simulink model "callGAMS"  (R2021b)
settings: Solver=ode1  StartTime=0.0  StopTime=20  FixedStep=1e-4  RelTol=1e-3
model workspace (MAT data in the model file):
  firstOrder = 60
  g2Max = 0
  runTime = 4
undefined symbols (not defined in the file or in its folder): c0, c1, D11, Delta, fg, G2gen, G3gen, G5gen, G6gen, G7gen, Iovc, l0, l1, Newton, r0, r1, Raphson, Rtpu, S1non, S2non, S3non, S5non, S6non, S7non, sigbuilder_block, tonvsc, Ts, Vhv, Vmv, w_pll, wc1, wdc1, wpq1, wsw1, Xtpu
libraries: simulink_extras x122, simulink x73, spsFirstOrderFilterLib x72, spsGroundLib x61, spsCurrentMeasurementLib x33, spsVoltageMeasurementLib x33, eeTransforms x24, spsabctoAlphaBetaZeroLib x12, spsControlledVoltageSourceLib x12, spsControlledCurrentSourceLib x12, spsPower3phPhasorLib x11, spsLoadFlowBusLib x9
(part 4 of 16)

== system callGAMS/sm_computation/G1/Speed Governor ==
  note: mechanical power
  RefL : Inport
  dw : Inport  Port=2
  Gain1 : Gain  Gain=Dt
  Gain2 : Gain  Gain=1/R
  Saturation : Saturate  UpperLimit=Vmax  LowerLimit=Vmin
  Saturation1 : Saturate  UpperLimit=1
  Sum : Sum  Inputs=|+-
  Sum1 : Sum  Inputs=|+-
  Transfer Fcn (with initial outputs)1 : simulink_extras/Additional Linear/Transfer Fcn (with initial outputs)  N=[T2 1]  D=[T3 1]  Y0=P0  U0=P0
  Transfer Fcn (with initial outputs)2 : simulink_extras/Additional Linear/Transfer Fcn (with initial outputs)  N=[1]  D=[T1 1]  Y0=P0  U0=P0
  Pm : Outport
  wires:
  Saturation1/1 -> Pm/1
  RefL/1 -> Sum/1
  Sum/1 -> Transfer Fcn (with initial outputs)2/1
  Transfer Fcn (with initial outputs)2/1 -> Saturation/1
  Saturation/1 -> Transfer Fcn (with initial outputs)1/1
  Sum1/1 -> Saturation1/1
  Transfer Fcn (with initial outputs)1/1 -> Sum1/1
  Gain1/1 -> Sum1/2
  dw/1 -> Gain1/1, Gain2/1
  Gain2/1 -> Sum/2

== system callGAMS/sm_computation/G2/G2 setpoint ==
  Clock : Clock
      settings: Decimation=runTime
  Clock1 : Clock
  Clock2 : Clock
      settings: Decimation=runTime
  Constant1 : Constant  Value=S2non*G2gen
  Constant2 : Constant  Value=S2non*G2gen
  Gain : Gain  Gain=1e6/1.2
  Gain1 : Gain  Gain=1/120
  Integrator : Integrator  InitialCondition=S2non*G2gen
  Memory : Memory
  Min : MinMax  Inputs=2
  Min1 : MinMax  Function=max  Inputs=2
  Sum : Sum  Inputs=|+-
  Sum1 : Sum
  Sum2 : Sum
  Sum3 : Sum
  Switch : Switch  Criteria=u2 > Threshold  Threshold=1  InputSameDT=on
  Switch1 : Switch  Criteria=u2 > Threshold  Threshold=runTime+1
  Switch2 : Switch  Criteria=u2 > Threshold  Threshold=runTime
  Switch3 : Switch  InputSameDT=on
  Switch4 : Switch  Criteria=u2 > Threshold  Threshold=runTime
  Out1 : Outport
  tag scope: g2Actual=global, g2Expected=global
  wires:
  [g2] -> Switch2/1
  Clock1/1 -> Switch1/2
  Sum1/1 -> Switch1/1
  Memory/1 -> Sum1/1
  Clock/1 -> Switch2/2
  Constant2/1 -> Switch2/3
  Switch/1 -> ?
  Gain/1 -> Sum2/2
  Switch2/1 -> Sum2/1, [g2Actual], Switch1/3
  [g2Reg] -> Sum1/2
  [g2Reg] -> Gain/1
  Sum2/1 -> Min1/2, Min/2
  Switch1/1 -> Switch/2, Switch/3, [A], Memory/1
  [A] -> Min1/1, Min/1
  [gSet] -> Switch/1
  [g2Reg] -> Switch3/2
  Min/1 -> Switch3/1
  Min1/1 -> Switch3/3
  Switch3/1 -> [gSet]
  [g2] -> Sum3/1
  Constant1/1 -> Switch4/3
  Clock2/1 -> Switch4/2
  Sum3/1 -> Switch4/1
  [g2Reg] -> Sum3/2
  Switch4/1 -> [g2Expected], Sum/1
  Integrator/1 -> Out1/1, Sum/2
  Sum/1 -> Gain1/1
  Gain1/1 -> Integrator/1

== system callGAMS/sm_computation/G2/VSC v2 ==
  note: If using different transformer connection,
      | compensate the delay in the modulation
  Pset : Inport
  Qset : Inport  Port=2
  Block : Step  Time=tonvsc  Before=1  After=0  SampleTime=0
  NOT : Logic  Operator=NOT  IconShape=distinctive  AllPortsSameDT=off  OutDataTypeStr=boolean
  Three-Phase Transformer (Two Windings)1 : spsThreePhaseTransformerTwoWindingsLib/Three-Phase Transformer (Two Windings)  Winding1Connection=Yg  Winding2Connection=Delta (D11)  CoreType=Three single-phase transformers  SetSaturation=off  Hysteresis=off  DataFile='hysteresis'  SetInitialFlux=off  Measurements=None  UNITS=pu  NominalPower=[Pconv , fg]  Winding1=[Vhv, Rtpu/2, Xtpu/2]  Winding2=[Vmv, Rtpu/2, Xtpu/2]  Rm=5000  Lm=5000  L0=0.5  Saturation=[ 0,0 ; 0.0024,1.2 ; 1.0,1.52 ]  InitialFluxes=[ 0.8 , -0.8 , 0.7 ]  BreakLoop=off  DiscreteSolver=Trapezoidal iterative  DataType=off  TransfoNumber=1
  VI measurement : Subsystem
  VSC Control : Subsystem
  VSC Model : Subsystem  Variant=on  VariantControlMode=label  LabelModeActiveChoice=Phasor
  output signals : Subsystem
  A : PMIOPort  Side=Left
  B : PMIOPort  Port=2  Side=Left
  C : PMIOPort  Port=3  Side=Left
  m : Outport
  tag scope: I2=global, V2=global
  wires:
  NOT/1 -> ?
  VSC Control/1(Ref) -> VSC Model/1(Ref)
  [Is] -> VSC Control/3(Iabc)
  Block/1 -> NOT/1, VSC Control/1(Block)
  [Vs] -> output signals/1(Vs)
  [Is] -> output signals/2(Is)
  VSC Control/2(m) -> output signals/3(control)
  output signals/1(m) -> m/1
  VI measurement/1(Vs) -> [V2], [Vs]
  VI measurement/2(Is) -> [I2], [Is]
  Qset/1 -> VSC Control/5(Qset)
  [Vs] -> VSC Control/2(Vabc)
  Pset/1 -> VSC Control/4(Pset)
  ? -> VSC Control/6(Edc)
  connections:
  Three-Phase Transformer (Two Windings)1/LConn3 -- VI measurement/LConn3
  Three-Phase Transformer (Two Windings)1/LConn2 -- VI measurement/LConn2
  Three-Phase Transformer (Two Windings)1/LConn1 -- VI measurement/LConn1
  Three-Phase Transformer (Two Windings)1/RConn3 -- VSC Model/LConn3
  Three-Phase Transformer (Two Windings)1/RConn2 -- VSC Model/LConn2
  Three-Phase Transformer (Two Windings)1/RConn1 -- VSC Model/LConn1
  VI measurement/RConn1 -- A/RConn1
  VI measurement/RConn2 -- B/RConn1
  VI measurement/RConn3 -- C/RConn1

== system callGAMS/sm_computation/G3/G3 setpoint ==
  Clock : Clock
      settings: Decimation=runTime
  Clock1 : Clock
  Clock2 : Clock
      settings: Decimation=runTime
  Constant1 : Constant  Value=S3non*G3gen
  Constant2 : Constant  Value=S3non*G3gen
  Gain : Gain  Gain=1e6/1.2
  Gain1 : Gain  Gain=1/120
  Integrator : Integrator  InitialCondition=S2non*G2gen
  Memory : Memory
  Min : MinMax  Inputs=2
  Min1 : MinMax  Function=max  Inputs=2
  Sum : Sum  Inputs=|+-
  Sum1 : Sum
  Sum2 : Sum
  Sum3 : Sum
  Switch : Switch  Criteria=u2 > Threshold  Threshold=1  InputSameDT=on
  Switch1 : Switch  Criteria=u2 > Threshold  Threshold=runTime+1
  Switch2 : Switch  Criteria=u2 > Threshold  Threshold=runTime
  Switch3 : Switch  InputSameDT=on
  Switch4 : Switch  Criteria=u2 > Threshold  Threshold=runTime
  Out1 : Outport
  tag scope: g3Expected=global, g3toOpt=global
  wires:
  [g3] -> Switch2/1
  Clock1/1 -> Switch1/2
  Sum1/1 -> Switch1/1
  Memory/1 -> Sum1/1
  Clock/1 -> Switch2/2
  Constant2/1 -> Switch2/3
  Switch/1 -> Out1/1
  Gain/1 -> Sum2/2
  Switch2/1 -> Switch1/3, [g3toOpt], Sum2/1
  [g3Reg] -> Sum1/2
  [g3Reg] -> Gain/1
  Sum2/1 -> Min1/2, Min/2
  Switch1/1 -> Memory/1, [A], Switch/3, Switch/2
  [A] -> Min1/1, Min/1
  [gSet] -> Switch/1
  [g3Reg] -> Switch3/2
  Min/1 -> Switch3/1
  Min1/1 -> Switch3/3
  Switch3/1 -> [gSet]
  Gain1/1 -> Integrator/1
  Sum/1 -> Gain1/1
  Integrator/1 -> Sum/2
  Sum3/1 -> Switch4/1
  Constant1/1 -> Switch4/3
  Clock2/1 -> Switch4/2
  [g3] -> Sum3/1
  [g3Reg] -> Sum3/2
  Switch4/1 -> [g3Expected], Sum/1

== system callGAMS/sm_computation/G3/VSC v2 ==
  note: If using different transformer connection,
      | compensate the delay in the modulation
  Pset : Inport
  Qset : Inport  Port=2
  Block : Step  Time=tonvsc  Before=1  After=0  SampleTime=0
  NOT : Logic  Operator=NOT  IconShape=distinctive  AllPortsSameDT=off  OutDataTypeStr=boolean
  Three-Phase Transformer (Two Windings) : spsThreePhaseTransformerTwoWindingsLib/Three-Phase Transformer (Two Windings)  Winding1Connection=Yg  Winding2Connection=Delta (D11)  CoreType=Three single-phase transformers  SetSaturation=off  Hysteresis=off  DataFile='hysteresis'  SetInitialFlux=off  Measurements=None  UNITS=pu  NominalPower=[Pconv , fg ]  Winding1=[Vhv, Rtpu/2, Xtpu/2]  Winding2=[Vmv, Rtpu/2, Xtpu/2]  Rm=5000  Lm=5000  L0=0.5  Saturation=[ 0,0 ; 0.0024,1.2 ; 1.0,1.52 ]  InitialFluxes=[ 0.8 , -0.8 , 0.7 ]  BreakLoop=off  DiscreteSolver=Trapezoidal iterative  DataType=off  TransfoNumber=1
  VI measurement1 : Subsystem
  VSC Control : Subsystem
  VSC Model : Subsystem  Variant=on  VariantControlMode=label  LabelModeActiveChoice=Phasor
  output signals : Subsystem
  A : PMIOPort  Side=Left
  B : PMIOPort  Port=2  Side=Left
  C : PMIOPort  Port=3  Side=Left
  m : Outport
  tag scope: I3=global, V3=global
  wires:
  NOT/1 -> ?
  VSC Control/1(Ref) -> VSC Model/1(Ref)
  [Is] -> VSC Control/3(Iabc)
  Block/1 -> NOT/1, VSC Control/1(Block)
  [Vs] -> output signals/1(Vs)
  [Is] -> output signals/2(Is)
  VSC Control/2(m) -> output signals/3(control)
  output signals/1(m) -> m/1
  VI measurement1/1(Vs) -> [V3], [Vs]
  VI measurement1/2(Is) -> [Is], [I3]
  Qset/1 -> VSC Control/5(Qset)
  [Vs] -> VSC Control/2(Vabc)
  ? -> VSC Control/6(Edc)
  Pset/1 -> VSC Control/4(Pset)
  connections:
  VI measurement1/LConn3 -- Three-Phase Transformer (Two Windings)/LConn3
  VI measurement1/LConn2 -- Three-Phase Transformer (Two Windings)/LConn2
  VI measurement1/LConn1 -- Three-Phase Transformer (Two Windings)/LConn1
  Three-Phase Transformer (Two Windings)/RConn3 -- VSC Model/LConn3
  Three-Phase Transformer (Two Windings)/RConn2 -- VSC Model/LConn2
  Three-Phase Transformer (Two Windings)/RConn1 -- VSC Model/LConn1
  VI measurement1/RConn1 -- A/RConn1
  VI measurement1/RConn2 -- B/RConn1
  VI measurement1/RConn3 -- C/RConn1

== system callGAMS/sm_computation/G5/G5 setpoint ==
  Clock : Clock
      settings: Decimation=runTime
  Clock1 : Clock
  Clock2 : Clock
      settings: Decimation=runTime
  Constant1 : Constant  Value=S5non*G5gen
  Constant2 : Constant  Value=S5non*G5gen
  Gain : Gain  Gain=1e6/1.2
  Gain1 : Gain  Gain=1/120
  Integrator : Integrator  InitialCondition=S2non*G2gen
  Memory : Memory
  Min : MinMax  Inputs=2
  Min1 : MinMax  Function=max  Inputs=2
  Sum : Sum  Inputs=|+-
  Sum1 : Sum
  Sum2 : Sum
  Sum3 : Sum
  Switch : Switch  Criteria=u2 > Threshold  Threshold=1  InputSameDT=on
  Switch1 : Switch  Criteria=u2 > Threshold  Threshold=runTime+1
  Switch2 : Switch  Criteria=u2 > Threshold  Threshold=runTime
  Switch3 : Switch  InputSameDT=on
  Switch4 : Switch  Criteria=u2 > Threshold  Threshold=runTime
  Out1 : Outport
  tag scope: g5Expected=global, g5toOpt=global
  wires:
  [g5] -> Switch2/1
  Clock1/1 -> Switch1/2
  Sum1/1 -> Switch1/1
  Memory/1 -> Sum1/1
  Clock/1 -> Switch2/2
  Constant2/1 -> Switch2/3
  Switch/1 -> Out1/1
  Gain/1 -> Sum2/2
  Switch2/1 -> Switch1/3, [g5toOpt], Sum2/1
  [g5Reg] -> Sum1/2
  [g5Reg] -> Gain/1
  Sum2/1 -> Min1/2, Min/2
  Switch1/1 -> Switch/2, Switch/3, [A], Memory/1
  [A] -> Min1/1, Min/1
  [gSet] -> Switch/1
  [g5Reg] -> Switch3/2
  Min/1 -> Switch3/1
  Min1/1 -> Switch3/3
  Switch3/1 -> [gSet]
  Gain1/1 -> Integrator/1
  Sum/1 -> Gain1/1
  Integrator/1 -> Sum/2
  Sum3/1 -> Switch4/1
  Constant1/1 -> Switch4/3
  Clock2/1 -> Switch4/2
  [g5] -> Sum3/1
  [g5Reg] -> Sum3/2
  Switch4/1 -> [g5Expected], Sum/1

== system callGAMS/sm_computation/G5/VSC v2 ==
  note: If using different transformer connection,
      | compensate the delay in the modulation
  Pset : Inport
  Qset : Inport  Port=2
  Block : Step  Time=tonvsc  Before=1  After=0  SampleTime=0
  NOT : Logic  Operator=NOT  IconShape=distinctive  AllPortsSameDT=off  OutDataTypeStr=boolean
  Three-Phase Transformer (Two Windings) : spsThreePhaseTransformerTwoWindingsLib/Three-Phase Transformer (Two Windings)  Winding1Connection=Yg  Winding2Connection=Delta (D11)  CoreType=Three single-phase transformers  SetSaturation=off  Hysteresis=off  DataFile='hysteresis'  SetInitialFlux=off  Measurements=None  UNITS=pu  NominalPower=[Pconv , fg]  Winding1=[Vhv, Rtpu/2, Xtpu/2]  Winding2=[Vmv, Rtpu/2, Xtpu/2]  Rm=5000  Lm=5000  L0=0.5  Saturation=[ 0,0 ; 0.0024,1.2 ; 1.0,1.52 ]  InitialFluxes=[ 0.8 , -0.8 , 0.7 ]  BreakLoop=off  DiscreteSolver=Trapezoidal iterative  DataType=off  TransfoNumber=1
  VI measurement1 : Subsystem
  VSC Control : Subsystem
  VSC Model : Subsystem  Variant=on  VariantControlMode=label  LabelModeActiveChoice=Phasor
  output signals : Subsystem
  A : PMIOPort  Side=Left
  B : PMIOPort  Port=2  Side=Left
  C : PMIOPort  Port=3  Side=Left
  m : Outport
  tag scope: I5=global, V5=global
  wires:
  NOT/1 -> ?
  VSC Control/1(Ref) -> VSC Model/1(Ref)
  [Is] -> VSC Control/3(Iabc)
  Block/1 -> NOT/1, VSC Control/1(Block)
  [Vs] -> output signals/1(Vs)
  [Is] -> output signals/2(Is)
  VSC Control/2(m) -> output signals/3(control)
  output signals/1(m) -> m/1
  VI measurement1/1(Vs) -> [V5], [Vs]
  VI measurement1/2(Is) -> [I5], [Is]
  Qset/1 -> VSC Control/5(Qset)
  [Vs] -> VSC Control/2(Vabc)
  ? -> VSC Control/6(Edc)
  Pset/1 -> VSC Control/4(Pset)
  connections:
  VI measurement1/LConn3 -- Three-Phase Transformer (Two Windings)/LConn3
  VI measurement1/LConn2 -- Three-Phase Transformer (Two Windings)/LConn2
  VI measurement1/LConn1 -- Three-Phase Transformer (Two Windings)/LConn1
  Three-Phase Transformer (Two Windings)/RConn3 -- VSC Model/LConn3
  Three-Phase Transformer (Two Windings)/RConn2 -- VSC Model/LConn2
  Three-Phase Transformer (Two Windings)/RConn1 -- VSC Model/LConn1
  VI measurement1/RConn1 -- A/RConn1
  B/RConn1 -- VI measurement1/RConn2
  C/RConn1 -- VI measurement1/RConn3

== system callGAMS/sm_computation/G6/G6 setpoint ==
  Clock : Clock
      settings: Decimation=runTime
  Clock1 : Clock
  Clock2 : Clock
      settings: Decimation=runTime
  Constant1 : Constant  Value=S6non*G6gen
  Constant2 : Constant  Value=S6non*G6gen
  Gain : Gain  Gain=1e6/1.2
  Gain1 : Gain  Gain=1/60
  Integrator : Integrator  InitialCondition=S6non*G6gen
  Memory : Memory
  Min : MinMax  Inputs=2
  Min1 : MinMax  Function=max  Inputs=2
  Sum : Sum  Inputs=|+-
  Sum1 : Sum
  Sum2 : Sum
  Sum3 : Sum
  Switch : Switch  Criteria=u2 > Threshold  Threshold=1  InputSameDT=on
  Switch1 : Switch  Criteria=u2 > Threshold  Threshold=runTime+1
  Switch2 : Switch  Criteria=u2 > Threshold  Threshold=runTime
  Switch3 : Switch  InputSameDT=on
  Switch4 : Switch  Criteria=u2 > Threshold  Threshold=runTime
  Out2 : Outport
  tag scope: g6Actual=global, g6Expected=global
  wires:
  [g6] -> Switch2/1
  Clock1/1 -> Switch1/2
  Sum1/1 -> Switch1/1
  Memory/1 -> Sum1/1
  Clock/1 -> Switch2/2
  Constant2/1 -> Switch2/3
  Switch/1 -> ?
  Gain/1 -> Sum2/2
  Switch2/1 -> Switch1/3, [g6Actual], Sum2/1
  [g6Reg] -> Sum1/2
  [g6Reg] -> Gain/1
  Sum2/1 -> Min1/2, Min/2
  Switch1/1 -> Switch/2, Switch/3, [A], Memory/1
  [A] -> Min1/1, Min/1
  [gSet] -> Switch/1
  [g6Reg] -> Switch3/2
  Min/1 -> Switch3/1
  Min1/1 -> Switch3/3
  Switch3/1 -> [gSet]
  Integrator/1 -> Out2/1, Sum/2
  Sum/1 -> Gain1/1
  Gain1/1 -> Integrator/1
  Constant1/1 -> Switch4/3
  [g6Reg] -> Sum3/2
  Sum3/1 -> Switch4/1
  Clock2/1 -> Switch4/2
  Switch4/1 -> [g6Expected], Sum/1
  [g6] -> Sum3/1

== system callGAMS/sm_computation/G6/VSC v2 ==
  note: If using different transformer connection,
      | compensate the delay in the modulation
  Pset : Inport
  Qset : Inport  Port=2
  Block : Step  Time=tonvsc  Before=1  After=0  SampleTime=0
  NOT : Logic  Operator=NOT  IconShape=distinctive  AllPortsSameDT=off  OutDataTypeStr=boolean
  Three-Phase Transformer (Two Windings) : spsThreePhaseTransformerTwoWindingsLib/Three-Phase Transformer (Two Windings)  Winding1Connection=Yg  Winding2Connection=Delta (D11)  CoreType=Three single-phase transformers  SetSaturation=off  Hysteresis=off  DataFile='hysteresis'  SetInitialFlux=off  Measurements=None  UNITS=pu  NominalPower=[Pconv , fg]  Winding1=[Vhv, Rtpu/2, Xtpu/2]  Winding2=[Vmv, Rtpu/2, Xtpu/2]  Rm=5000  Lm=5000  L0=0.5  Saturation=[ 0,0 ; 0.0024,1.2 ; 1.0,1.52 ]  InitialFluxes=[ 0.8 , -0.8 , 0.7 ]  BreakLoop=off  DiscreteSolver=Trapezoidal iterative  DataType=off  TransfoNumber=1
  VI measurement1 : Subsystem
  VSC Control : Subsystem
  VSC Model : Subsystem  Variant=on  VariantControlMode=label  LabelModeActiveChoice=Phasor
  output signals : Subsystem
  A : PMIOPort  Side=Left
  B : PMIOPort  Port=2  Side=Left
  C : PMIOPort  Port=3  Side=Left
  m : Outport
  tag scope: I6=global, V6=global
  wires:
  NOT/1 -> ?
  VSC Control/1(Ref) -> VSC Model/1(Ref)
  [Is] -> VSC Control/3(Iabc)
  Block/1 -> NOT/1, VSC Control/1(Block)
  [Vs] -> output signals/1(Vs)
  [Is] -> output signals/2(Is)
  VSC Control/2(m) -> output signals/3(control)
  output signals/1(m) -> m/1
  VI measurement1/1(Vs) -> [V6], [Vs]
  VI measurement1/2(Is) -> [I6], [Is]
  Qset/1 -> VSC Control/5(Qset)
  [Vs] -> VSC Control/2(Vabc)
  ? -> VSC Control/6(Edc)
  Pset/1 -> VSC Control/4(Pset)
  connections:
  VI measurement1/LConn3 -- Three-Phase Transformer (Two Windings)/LConn3
  VI measurement1/LConn2 -- Three-Phase Transformer (Two Windings)/LConn2
  VI measurement1/LConn1 -- Three-Phase Transformer (Two Windings)/LConn1
  Three-Phase Transformer (Two Windings)/RConn3 -- VSC Model/LConn3
  Three-Phase Transformer (Two Windings)/RConn2 -- VSC Model/LConn2
  VI measurement1/RConn1 -- A/RConn1
  VI measurement1/RConn2 -- B/RConn1
  VI measurement1/RConn3 -- C/RConn1
  VSC Model/LConn1 -- Three-Phase Transformer (Two Windings)/RConn1

== system callGAMS/sm_computation/G7/Exciter System ==
  <dw> : Inport
  Vref : Inport  Port=2
  Vt : Inport  Port=3
  It : Inport  Port=4
  <Peo> : Inport  Port=5
  PSS1 : Subsystem  mask{Ks1=20, Ks2=0.1564, Ks3=1, Tw1=2, Tw2=2, Tw3=2, Tw4=0, T1=0.25, T2=0.2, T3=0.15, T4=0.1, T6=0, T7=2, T8=0.5, T9=0.1, Vstmin=-0.10, Vstmax=0.10, N=0, M=0, IC1=1, IC2=3}
      mask prompts: Ks1 "PSS gain (Ks1)"; Ks2 "2nd signal transducer factor(Ks2)"; Ks3 "washouts coupling factor (Ks3)"; Tw1 "1st washout 1th time constant (Tw1)(sec)"; Tw2 "1st washout 2nd time constant (Tw2)(sec)"; Tw3 "2nd washout 1st time constant (Tw3)(sec)"; Tw4 "2nd washout 2nd time constant (Tw4)(sec)"; T1 "1st lead-lag derivative time constant (T1)(sec)"; T2 "1st lead-lag delay time constant(T2)(sec)"; T3 "2nd lead-lag derivative time constant(T3)(sec)"; T4 "2nd lead-lag delay time constant(T4)(sec)"; T6 "1st signal transducer time constant(T6)(sec)"; T7 "2nd signal transducer time constant(T7)(sec)"; T8 "ramp tracking filter deriv. time constant(T8)(sec)"; T9 "ramp tracking filter delay time constant(T9)(sec)"; Vstmin "controller minimum output(Vstmin)"; Vstmax "controller maximum output(Vstmax)"; N "ramp tracking filter (N)"; M "ramp tracking filter (M)"; IC1 "1st input selector (IC1)"; IC2 "2nd input selector (IC2)"
      mask Display:
      | disp('PSS2A')
      | 
      | port_label('input',1,'dw')
      | port_label('input',2,'Pg')
      | %port_label('input',3,'Vs')
      | 
      | port_label('output',1,'Vs')
  SEXS : Subsystem  mask{K=200, Ta=3, Tb=10, Te=0.05, Emin=-4, Emax=4, Vf0=1.3543}
      mask prompts: K "Controller gain (K)"; Ta "Filter derivative time constant (Ta)(sec)"; Tb "Filter delay time (Tb)(sec)"; Te "Exciter time constant (Te)(sec)"; Emin "Controller minimum output (Emin)"; Emax "Controller maximum output (Emax)"; Vf0 "Initial output (p.u)"
      mask Display:
      | disp('AVR')
      | 
      | port_label('input',1,'Vref')
      | port_label('input',2,'Vc')
      | port_label('input',3,'Vs')
      | 
      | port_label('output',1,'Efd')
  TR and LC_test : Subsystem  mask{Tr=1e-3, Rc=0, Xc=0}
      mask prompts: Tr "Transducter filter time constant (Tr)(sec)"; Rc "Resistance to compensate (p.u)"; Xc "Reactance to compensate (p.u)"
      mask Display:
      | %disp('Transducer \n \n')
      | %disp('and \n')
      | %disp('Load compensation')
      | text(15,35, 'Transducer')
      | text(30,24, 'and')
      | text(15,14, 'Load comp')
      | 
      | port_label('input',1,'Vt')
      | port_label('input',2,'It')
      | 
      | port_label('output',1,'Vc')
  Efd : Outport
  wires:
  TR and LC_test/1(Vc) -> SEXS/2(Vc)
  Vref/1 -> SEXS/1(Vref)
  Vt/1 -> TR and LC_test/1(Vt)
  <dw>/1 -> PSS1/1(dw)
  <Peo>/1 -> PSS1/2(Pgen)
  PSS1/1(Vothsg) -> SEXS/3(Vs)
  It/1 -> TR and LC_test/2(It)
  SEXS/1(Efd) -> Efd/1

== system callGAMS/sm_computation/G7/Speed Governor ==
  note: mechanical power
  RefL : Inport
  dw : Inport  Port=2
  Gain1 : Gain  Gain=Dt
  Gain2 : Gain  Gain=1/R
  Saturation : Saturate  UpperLimit=Vmax  LowerLimit=Vmin
  Saturation1 : Saturate  UpperLimit=1
  Sum : Sum  Inputs=|+-
  Sum1 : Sum  Inputs=|+-
  Transfer Fcn (with initial outputs)1 : simulink_extras/Additional Linear/Transfer Fcn (with initial outputs)  N=[T2 1]  D=[T3 1]  Y0=P0  U0=P0
  Transfer Fcn (with initial outputs)2 : simulink_extras/Additional Linear/Transfer Fcn (with initial outputs)  N=[1]  D=[T1 1]  Y0=P0  U0=P0
  Pm : Outport
  wires:
  Saturation1/1 -> Pm/1
  RefL/1 -> Sum/1
  Sum/1 -> Transfer Fcn (with initial outputs)2/1
  Transfer Fcn (with initial outputs)2/1 -> Saturation/1
  Saturation/1 -> Transfer Fcn (with initial outputs)1/1
  Sum1/1 -> Saturation1/1
  Transfer Fcn (with initial outputs)1/1 -> Sum1/1
  Gain1/1 -> Sum1/2
  dw/1 -> Gain1/1, Gain2/1
  Gain2/1 -> Sum/2

== system callGAMS/sm_computation/Measurements EMT/Subsystem ==
  In1 : Inport
  Gain : Gain  Gain=1/3
  Mean value : spsMeanLib/Mean  Freq=fg  Vinit=Vrms0  Ts=Ts
  Product : Product  InputSameDT=on  SaturateOnIntegerOverflow=on  OutDataTypeStr=Inherit: Same as first input
  Saturation to avoid negative sqrt : Saturate  UpperLimit=Inf  LowerLimit=0
  Sqrt : Sqrt  AlgorithmType=Newton-Raphson  SaturateOnIntegerOverflow=on
  Sum of Elements : Sum  Inputs=+
  Out1 : Outport
  wires:
  Sqrt/1 -> Sum of Elements/1
  Mean value/1 -> Saturation to avoid negative sqrt/1
  Saturation to avoid negative sqrt/1 -> Sqrt/1
  Product/1 -> Mean value/1
  In1/1 -> Product/2, Product/1
  Sum of Elements/1 -> Gain/1
  Gain/1 -> Out1/1

== system callGAMS/sm_computation/Measurements EMT/Subsystem1 ==
  In1 : Inport
  Gain : Gain  Gain=1/3
  Mean value : spsMeanLib/Mean  Freq=fg  Vinit=Vrms0  Ts=Ts
  Product : Product  InputSameDT=on  SaturateOnIntegerOverflow=on  OutDataTypeStr=Inherit: Same as first input
  Saturation to avoid negative sqrt : Saturate  UpperLimit=Inf  LowerLimit=0
  Sqrt : Sqrt  AlgorithmType=Newton-Raphson  SaturateOnIntegerOverflow=on
  Sum of Elements : Sum  Inputs=+
  Out1 : Outport
  wires:
  Sqrt/1 -> Sum of Elements/1
  Mean value/1 -> Saturation to avoid negative sqrt/1
  Saturation to avoid negative sqrt/1 -> Sqrt/1
  Product/1 -> Mean value/1
  In1/1 -> Product/2, Product/1
  Sum of Elements/1 -> Gain/1
  Gain/1 -> Out1/1

== system callGAMS/sm_computation/Measurements EMT/Subsystem2 ==
  In1 : Inport
  Gain : Gain  Gain=1/3
  Mean value : spsMeanLib/Mean  Freq=fg  Vinit=Vrms0  Ts=Ts
  Product : Product  InputSameDT=on  SaturateOnIntegerOverflow=on  OutDataTypeStr=Inherit: Same as first input
  Saturation to avoid negative sqrt : Saturate  UpperLimit=Inf  LowerLimit=0
  Sqrt : Sqrt  AlgorithmType=Newton-Raphson  SaturateOnIntegerOverflow=on
  Sum of Elements : Sum  Inputs=+
  Out1 : Outport
  wires:
  Sqrt/1 -> Sum of Elements/1
  Mean value/1 -> Saturation to avoid negative sqrt/1
  Saturation to avoid negative sqrt/1 -> Sqrt/1
  Product/1 -> Mean value/1
  In1/1 -> Product/2, Product/1
  Sum of Elements/1 -> Gain/1
  Gain/1 -> Out1/1

== system callGAMS/sm_computation/Measurements EMT/Subsystem3 ==
  In1 : Inport
  Gain : Gain  Gain=1/3
  Mean value : spsMeanLib/Mean  Freq=fg  Vinit=Vrms0  Ts=Ts
  Product : Product  InputSameDT=on  SaturateOnIntegerOverflow=on  OutDataTypeStr=Inherit: Same as first input
  Saturation to avoid negative sqrt : Saturate  UpperLimit=Inf  LowerLimit=0
  Sqrt : Sqrt  AlgorithmType=Newton-Raphson  SaturateOnIntegerOverflow=on
  Sum of Elements : Sum  Inputs=+
  Out1 : Outport
  wires:
  Sqrt/1 -> Sum of Elements/1
  Mean value/1 -> Saturation to avoid negative sqrt/1
  Saturation to avoid negative sqrt/1 -> Sqrt/1
  Product/1 -> Mean value/1
  In1/1 -> Product/2, Product/1
  Sum of Elements/1 -> Gain/1
  Gain/1 -> Out1/1

== system callGAMS/sm_computation/Measurements EMT/Subsystem4 ==
  In1 : Inport
  Gain : Gain  Gain=1/3
  Mean value : spsMeanLib/Mean  Freq=fg  Vinit=Vrms0  Ts=Ts
  Product : Product  InputSameDT=on  SaturateOnIntegerOverflow=on  OutDataTypeStr=Inherit: Same as first input
  Saturation to avoid negative sqrt : Saturate  UpperLimit=Inf  LowerLimit=0
  Sqrt : Sqrt  AlgorithmType=Newton-Raphson  SaturateOnIntegerOverflow=on
  Sum of Elements : Sum  Inputs=+
  Out1 : Outport
  wires:
  Sqrt/1 -> Sum of Elements/1
  Mean value/1 -> Saturation to avoid negative sqrt/1
  Saturation to avoid negative sqrt/1 -> Sqrt/1
  Product/1 -> Mean value/1
  In1/1 -> Product/2, Product/1
  Sum of Elements/1 -> Gain/1
  Gain/1 -> Out1/1

== system callGAMS/sm_computation/Measurements EMT/Subsystem5 ==
  In1 : Inport
  Gain : Gain  Gain=1/3
  Mean value : spsMeanLib/Mean  Freq=fg  Vinit=Vrms0  Ts=Ts
  Product : Product  InputSameDT=on  SaturateOnIntegerOverflow=on  OutDataTypeStr=Inherit: Same as first input
  Saturation to avoid negative sqrt : Saturate  UpperLimit=Inf  LowerLimit=0
  Sqrt : Sqrt  AlgorithmType=Newton-Raphson  SaturateOnIntegerOverflow=on
  Sum of Elements : Sum  Inputs=+
  Out1 : Outport
  wires:
  Sqrt/1 -> Sum of Elements/1
  Mean value/1 -> Saturation to avoid negative sqrt/1
  Saturation to avoid negative sqrt/1 -> Sqrt/1
  Product/1 -> Mean value/1
  In1/1 -> Product/2, Product/1
  Sum of Elements/1 -> Gain/1
  Gain/1 -> Out1/1

== system callGAMS/sm_computation/Measurements Phasor/Subsystem1 ==
  abc : Inport
  Gain1 : Gain  Gain=[1 a a2]  SaturateOnIntegerOverflow=on  OutDataTypeStr=Inherit: Same as input  ParamDataTypeStr=Inherit: Same as input
  Gain3 : Gain  Gain=1/3  SaturateOnIntegerOverflow=on  OutDataTypeStr=Inherit: Same as input  ParamDataTypeStr=Inherit: Same as input
  Sum : Sum  Inputs=1  InputSameDT=on  SaturateOnIntegerOverflow=on  OutDataTypeStr=Inherit: Same as first input
  seq+ : Outport
  wires:
  Sum/1 -> Gain3/1
  abc/1 -> Gain1/1
  Gain1/1 -> Sum/1
  Gain3/1 -> seq+/1

== system callGAMS/sm_computation/Measurements Phasor/Subsystem2 ==
  abc : Inport
  Gain1 : Gain  Gain=[1 a a2]  SaturateOnIntegerOverflow=on  OutDataTypeStr=Inherit: Same as input  ParamDataTypeStr=Inherit: Same as input
  Gain3 : Gain  Gain=1/3  SaturateOnIntegerOverflow=on  OutDataTypeStr=Inherit: Same as input  ParamDataTypeStr=Inherit: Same as input
  Sum : Sum  Inputs=1  InputSameDT=on  SaturateOnIntegerOverflow=on  OutDataTypeStr=Inherit: Same as first input
  seq+ : Outport
  wires:
  Gain3/1 -> seq+/1
  Gain1/1 -> Sum/1
  abc/1 -> Gain1/1
  Sum/1 -> Gain3/1

== system callGAMS/sm_computation/Measurements Phasor/Subsystem3 ==
  abc : Inport
  Gain1 : Gain  Gain=[1 a a2]  SaturateOnIntegerOverflow=on  OutDataTypeStr=Inherit: Same as input  ParamDataTypeStr=Inherit: Same as input
  Gain3 : Gain  Gain=1/3  SaturateOnIntegerOverflow=on  OutDataTypeStr=Inherit: Same as input  ParamDataTypeStr=Inherit: Same as input
  Sum : Sum  Inputs=1  InputSameDT=on  SaturateOnIntegerOverflow=on  OutDataTypeStr=Inherit: Same as first input
  seq+ : Outport
  wires:
  Gain3/1 -> seq+/1
  Gain1/1 -> Sum/1
  abc/1 -> Gain1/1
  Sum/1 -> Gain3/1

== system callGAMS/sm_computation/Measurements Phasor/Subsystem4 ==
  abc : Inport
  Gain1 : Gain  Gain=[1 a a2]  SaturateOnIntegerOverflow=on  OutDataTypeStr=Inherit: Same as input  ParamDataTypeStr=Inherit: Same as input
  Gain3 : Gain  Gain=1/3  SaturateOnIntegerOverflow=on  OutDataTypeStr=Inherit: Same as input  ParamDataTypeStr=Inherit: Same as input
  Sum : Sum  Inputs=1  InputSameDT=on  SaturateOnIntegerOverflow=on  OutDataTypeStr=Inherit: Same as first input
  seq+ : Outport
  wires:
  Sum/1 -> Gain3/1
  abc/1 -> Gain1/1
  Gain1/1 -> Sum/1
  Gain3/1 -> seq+/1

== system callGAMS/sm_computation/Measurements Phasor/Subsystem5 ==
  abc : Inport
  Gain1 : Gain  Gain=[1 a a2]  SaturateOnIntegerOverflow=on  OutDataTypeStr=Inherit: Same as input  ParamDataTypeStr=Inherit: Same as input
  Gain3 : Gain  Gain=1/3  SaturateOnIntegerOverflow=on  OutDataTypeStr=Inherit: Same as input  ParamDataTypeStr=Inherit: Same as input
  Sum : Sum  Inputs=1  InputSameDT=on  SaturateOnIntegerOverflow=on  OutDataTypeStr=Inherit: Same as first input
  seq+ : Outport
  wires:
  Gain3/1 -> seq+/1
  Gain1/1 -> Sum/1
  abc/1 -> Gain1/1
  Sum/1 -> Gain3/1

== system callGAMS/sm_computation/Measurements Phasor/Subsystem6 ==
  abc : Inport
  Gain1 : Gain  Gain=[1 a a2]  SaturateOnIntegerOverflow=on  OutDataTypeStr=Inherit: Same as input  ParamDataTypeStr=Inherit: Same as input
  Gain3 : Gain  Gain=1/3  SaturateOnIntegerOverflow=on  OutDataTypeStr=Inherit: Same as input  ParamDataTypeStr=Inherit: Same as input
  Sum : Sum  Inputs=1  InputSameDT=on  SaturateOnIntegerOverflow=on  OutDataTypeStr=Inherit: Same as first input
  seq+ : Outport
  wires:
  Sum/1 -> Gain3/1
  abc/1 -> Gain1/1
  Gain1/1 -> Sum/1
  Gain3/1 -> seq+/1

== system callGAMS/sm_computation/G1/Exciter System/PSS1 ==
  note: Power System Stabilizer (PSS2A)
  dw : Inport
  Pgen : Inport  Port=2
  Gain : Gain  Gain=Ks1
  Gain1 : Gain  Gain=Ks3
  Saturation : Saturate  UpperLimit=Vstmax  LowerLimit=Vstmin
  Sum1 : Sum  Inputs=|++
  Sum2 : Sum  Inputs=|+-
  Transfer Fcn1 : TransferFcn  Numerator=[Tw1 0]  Denominator=[Tw1 1]
  Transfer Fcn2 : TransferFcn  Numerator=[Tw3 0]  Denominator=[Tw3 1]
  Transfer Fcn3 : TransferFcn  Numerator=[Tw2 0]  Denominator=[Tw2 1]
  Transfer Fcn4 : TransferFcn  Denominator=[T6 1]
  Transfer Fcn5 : TransferFcn  Numerator=[T8 1].^N  Denominator=[T9 1].^(M*N)
  Transfer Fcn6 : TransferFcn  Numerator=[T1 1]  Denominator=[T2 1]
  Transfer Fcn7 : TransferFcn  Numerator=[T3 1]  Denominator=[T4 1]
  Transfer Fcn8 : TransferFcn  Numerator=[Tw4 0]  Denominator=[Tw4 1]
  Transfer Fcn9 : TransferFcn  Numerator=[Ks2]  Denominator=[T7 1]
  Vothsg : Outport
  wires:
  dw/1 -> Transfer Fcn1/1
  Transfer Fcn1/1 -> Transfer Fcn3/1
  Transfer Fcn3/1 -> Transfer Fcn4/1
  Transfer Fcn4/1 -> Sum1/1
  Sum1/1 -> Transfer Fcn5/1
  Transfer Fcn5/1 -> Sum2/1
  Sum2/1 -> Gain/1
  Gain/1 -> Transfer Fcn6/1
  Transfer Fcn6/1 -> Transfer Fcn7/1
  Transfer Fcn7/1 -> Saturation/1
  Saturation/1 -> Vothsg/1
  Pgen/1 -> Transfer Fcn2/1
  Transfer Fcn2/1 -> Transfer Fcn8/1
  Transfer Fcn8/1 -> Transfer Fcn9/1
  Gain1/1 -> Sum1/2
  Transfer Fcn9/1 -> Gain1/1, Sum2/2

== system callGAMS/sm_computation/G1/Exciter System/SEXS ==
  note: The controller parameters provided by ENTSO-E
      | define different names for the parameters:
      |
      | ENTSO-E = IEEE Std 421.5-2005
      | Ta = Tc
      | Tb = Tb
      | K = Ka
      | Te = Ta
      | Emax = Vrmax
      | Emin = Vrmin
  note: The exciter model provided by ENTSO-E most similar to the IEEE is the Type AC4A excitation system model
  Vref : Inport
  Vc : Inport  Port=2
  Vs : Inport  Port=3
  1st ord transfer fcn windup limiter : Subsystem  mask{Gain=K, tau=Te, Vmax=Emax, Vmin=Emin, y0=Vf0}
      mask prompts: tau "Time constant"; y0 "Initial output"
  Constant : Constant  Value=Vf0/K
  Saturation : Saturate  Commented=through  UpperLimit=0.1  LowerLimit=-0.1
  Sum : Sum  Inputs=+-+
  Sum1 : Sum  Inputs=|++
  Transfer Fcn (with initial outputs)1 : simulink_extras/Additional Linear/Transfer Fcn (with initial outputs)  N=[Ta 1]  D=[Tb 1]  Y0=Vf0/K  U0=Vf0/K
  Efd : Outport
  wires:
  1st ord transfer fcn windup limiter/1(Out1) -> Efd/1
  Vs/1 -> Sum/3
  Vref/1 -> Sum/1
  Vc/1 -> Sum/2
  Transfer Fcn (with initial outputs)1/1 -> 1st ord transfer fcn windup limiter/1(In1)
  Saturation/1 -> Transfer Fcn (with initial outputs)1/1
  Sum/1 -> Sum1/1
  Sum1/1 -> Saturation/1
  Constant/1 -> Sum1/2

== system callGAMS/sm_computation/G1/Exciter System/TR and LC_test ==
  note: Terminal voltage transducer and optional load compensation
  note: compensated
      | impedance
  note: Vt and It should be phasors (complex quantities)
  note: Fig 4.1 of IEEE Std 421.5-2005
  note: Rc and Xc should be negative values in case of voltage regulated after an impedance
  Vt : Inport
  It : Inport  Port=2
  Abs : Abs
  Abs1 : Abs
  Rc+jXc : Gain  Gain=abs(Rc+1i*Xc)
  Saturation : Saturate  UpperLimit=1.2  LowerLimit=0.8
  Sum : Sum  Inputs=|+-
  Transfer Fcn (with initial outputs) : simulink_extras/Additional Linear/Transfer Fcn (with initial outputs)  Commented=through  N=[1]  D=[Tr 1]  Y0=1  U0=1
  Vc : Outport
  wires:
  Saturation/1 -> Vc/1
  Vt/1 -> Abs/1
  Transfer Fcn (with initial outputs)/1 -> Saturation/1
  Rc+jXc/1 -> Sum/2
  Sum/1 -> Transfer Fcn (with initial outputs)/1
  It/1 -> Abs1/1
  Abs/1 -> Sum/1
  Abs1/1 -> Rc+jXc/1

== system callGAMS/sm_computation/G2/VSC v2/VI measurement ==
  Current Measurement : spsCurrentMeasurementLib/Current Measurement  PhasorSimulation=on  OutputType=Complex  PSBequivalent=0
  Current Measurement1 : spsCurrentMeasurementLib/Current Measurement  PhasorSimulation=on  OutputType=Complex  PSBequivalent=0
  Current Measurement2 : spsCurrentMeasurementLib/Current Measurement  PhasorSimulation=on  OutputType=Complex  PSBequivalent=0
  Ground : spsGroundLib/Ground  LConnTagsString=a
  Ground1 : spsGroundLib/Ground  LConnTagsString=a
  Ground2 : spsGroundLib/Ground  LConnTagsString=a
  Mux : Mux  Inputs=3
  Mux1 : Mux  Inputs=3
  Voltage Measurement1 : spsVoltageMeasurementLib/Voltage Measurement  PhasorSimulation=on  OutputType=Complex  PSBequivalent=0
  Voltage Measurement2 : spsVoltageMeasurementLib/Voltage Measurement  PhasorSimulation=on  OutputType=Complex  PSBequivalent=0
  Voltage Measurement3 : spsVoltageMeasurementLib/Voltage Measurement  PhasorSimulation=on  OutputType=Complex  PSBequivalent=0
  A : PMIOPort  Side=Left
  B : PMIOPort  Port=2  Side=Left
  C : PMIOPort  Port=3  Side=Left
  a : PMIOPort  Port=4  Side=Right
  b : PMIOPort  Port=5  Side=Right
  c : PMIOPort  Port=6  Side=Right
  Vs : Outport
  Is : Outport  Port=2
  wires:
  Mux1/1 -> Is/1
  Mux/1 -> Vs/1
  Voltage Measurement1/1 -> Mux/2
  Voltage Measurement2/1 -> Mux/3
  Current Measurement2/1 -> Mux1/3
  Voltage Measurement3/1 -> Mux/1
  Current Measurement/1 -> Mux1/1
  Current Measurement1/1 -> Mux1/2
  connections:
  Current Measurement/LConn1 -- Voltage Measurement3/LConn1 -- A/RConn1
  C/RConn1 -- Current Measurement2/LConn1 -- Voltage Measurement2/LConn1
  Voltage Measurement1/LConn1 -- Current Measurement1/LConn1 -- B/RConn1
  Current Measurement1/RConn1 -- b/RConn1
  Current Measurement/RConn1 -- a/RConn1
  Current Measurement2/RConn1 -- c/RConn1
  Ground1/LConn1 -- Voltage Measurement1/LConn2
  Ground2/LConn1 -- Voltage Measurement2/LConn2
  Voltage Measurement3/LConn2 -- Ground/LConn1

== system callGAMS/sm_computation/G2/VSC v2/VSC Control ==
  Block : Inport
  Vabc : Inport  Port=2
  Iabc : Inport  Port=3
  Pset : Inport  Port=4
  Qset : Inport  Port=5
  Edc : Inport  Port=6
  Control loops : Subsystem  Variant=on  VariantControlMode=label  LabelModeActiveChoice=Phasor_I_ref
  Measurements : Subsystem  Variant=on  VariantControlMode=label  LabelModeActiveChoice=Phasor
  Modulation : Subsystem  Variant=on  VariantControlMode=label  LabelModeActiveChoice=Phasor_I_and_PQ
  Mux : Mux  Inputs=2
  Ref : Outport
  m : Outport  Port=2
  wires:
  Control loops/2(iqd+-ref) -> Modulation/3(iqd+-*)
  Control loops/1(vqd+-ref) -> Modulation/2(vqd+-*)
  [PQabc] -> Mux/2
  Measurements/5(PQabc) -> [PQabc]
  Modulation/1(Ref) -> Ref/1
  Measurements/4(theta) -> [theta]
  Vabc/1 -> Measurements/1(Vabc)
  Measurements/1(vqd+-) -> Control loops/3(vqd+-), [vqdpn]
  Measurements/2(iqd+-) -> Control loops/4(iqd+-)
  Measurements/3(freq) -> Control loops/5(freq)
  [theta] -> Modulation/4(theta)
  [vqdpn] -> Modulation/1(vqd+-)
  Iabc/1 -> Measurements/2(Iabc)
  Mux/1 -> m/1
  Control loops/3(m) -> Mux/1
  Pset/1 -> Control loops/1(Pset)
  Qset/1 -> Control loops/2(Qset)
  Block/1 -> Control loops/6(Block)
  Edc/1 -> Control loops/7(Edc)

== system callGAMS/sm_computation/G2/VSC v2/VSC Model ==
  Ref : Inport
  EMT AVG : Subsystem  VariantControl=EMT_AVG
  EMT SW : Subsystem  VariantControl=EMT_SW
  Phasor : Subsystem  VariantControl=Phasor
  A : PMIOPort  Side=Left
  B : PMIOPort  Port=2  Side=Left
  C : PMIOPort  Port=3  Side=Left

== system callGAMS/sm_computation/G2/VSC v2/output signals ==
  Vs : Inport
  Is : Inport  Port=2
  control : Inport  Port=3
  Bus Creator : BusCreator  Inputs=15
  Demux : Demux  Outputs=13
  m : Outport
  wires:
  Bus Creator/1 -> m/1
  control/1 -> Demux/1
  Vs/1 -> Bus Creator/1  "Vabc"
  Is/1 -> Bus Creator/2  "Iabc"
  Demux/1 -> Bus Creator/3  "vqp"
  Demux/2 -> Bus Creator/4  "vdp"
  Demux/3 -> Bus Creator/5  "vqn"
  Demux/4 -> Bus Creator/6  "vdn"
  Demux/5 -> Bus Creator/7  "iqp"
  Demux/6 -> Bus Creator/8  "idp"
  Demux/7 -> Bus Creator/9  "iqn"
  Demux/8 -> Bus Creator/10  "idn"
  Demux/9 -> Bus Creator/11  "f"
  Demux/10 -> Bus Creator/12  "Pdq"
  Demux/11 -> Bus Creator/13  "Qdq"
  Demux/12 -> Bus Creator/14  "Pabc"
  Demux/13 -> Bus Creator/15  "Qabc"

== system callGAMS/sm_computation/G3/VSC v2/VI measurement1 ==
  Current Measurement : spsCurrentMeasurementLib/Current Measurement  PhasorSimulation=on  OutputType=Complex  PSBequivalent=0
  Current Measurement1 : spsCurrentMeasurementLib/Current Measurement  PhasorSimulation=on  OutputType=Complex  PSBequivalent=0
  Current Measurement2 : spsCurrentMeasurementLib/Current Measurement  PhasorSimulation=on  OutputType=Complex  PSBequivalent=0
  Ground : spsGroundLib/Ground  LConnTagsString=a
  Ground1 : spsGroundLib/Ground  LConnTagsString=a
  Ground2 : spsGroundLib/Ground  LConnTagsString=a
  Mux : Mux  Inputs=3
  Mux1 : Mux  Inputs=3
  Voltage Measurement1 : spsVoltageMeasurementLib/Voltage Measurement  PhasorSimulation=on  OutputType=Complex  PSBequivalent=0
  Voltage Measurement2 : spsVoltageMeasurementLib/Voltage Measurement  PhasorSimulation=on  OutputType=Complex  PSBequivalent=0
  Voltage Measurement3 : spsVoltageMeasurementLib/Voltage Measurement  PhasorSimulation=on  OutputType=Complex  PSBequivalent=0
  A : PMIOPort  Side=Left
  B : PMIOPort  Port=2  Side=Left
  C : PMIOPort  Port=3  Side=Left
  a : PMIOPort  Port=4  Side=Right
  b : PMIOPort  Port=5  Side=Right
  c : PMIOPort  Port=6  Side=Right
  Vs : Outport
  Is : Outport  Port=2
  wires:
  Mux1/1 -> Is/1
  Mux/1 -> Vs/1
  Voltage Measurement1/1 -> Mux/2
  Voltage Measurement2/1 -> Mux/3
  Current Measurement2/1 -> Mux1/3
  Voltage Measurement3/1 -> Mux/1
  Current Measurement/1 -> Mux1/1
  Current Measurement1/1 -> Mux1/2
  connections:
  Voltage Measurement3/LConn1 -- A/RConn1 -- Current Measurement/LConn1
  Current Measurement2/LConn1 -- C/RConn1 -- Voltage Measurement2/LConn1
  B/RConn1 -- Voltage Measurement1/LConn1 -- Current Measurement1/LConn1
  Current Measurement1/RConn1 -- b/RConn1
  Current Measurement/RConn1 -- a/RConn1
  Current Measurement2/RConn1 -- c/RConn1
  Ground2/LConn1 -- Voltage Measurement2/LConn2
  Ground/LConn1 -- Voltage Measurement3/LConn2
  Ground1/LConn1 -- Voltage Measurement1/LConn2

== system callGAMS/sm_computation/G3/VSC v2/VSC Control ==
  Block : Inport
  Vabc : Inport  Port=2
  Iabc : Inport  Port=3
  Pset : Inport  Port=4
  Qset : Inport  Port=5
  Edc : Inport  Port=6
  Control loops : Subsystem  Variant=on  VariantControlMode=label  LabelModeActiveChoice=Phasor_I_ref
  Measurements : Subsystem  Variant=on  VariantControlMode=label  LabelModeActiveChoice=Phasor
  Modulation : Subsystem  Variant=on  VariantControlMode=label  LabelModeActiveChoice=Phasor_I_and_PQ
  Mux : Mux  Inputs=2
  Ref : Outport
  m : Outport  Port=2
  wires:
  Control loops/2(iqd+-ref) -> Modulation/3(iqd+-*)
  Control loops/1(vqd+-ref) -> Modulation/2(vqd+-*)
  [PQabc] -> Mux/2
  Measurements/5(PQabc) -> [PQabc]
  Modulation/1(Ref) -> Ref/1
  Measurements/4(theta) -> [theta]
  Vabc/1 -> Measurements/1(Vabc)
  Measurements/1(vqd+-) -> Control loops/3(vqd+-), [vqdpn]
  Measurements/2(iqd+-) -> Control loops/4(iqd+-)
  Measurements/3(freq) -> Control loops/5(freq)
  [theta] -> Modulation/4(theta)
  [vqdpn] -> Modulation/1(vqd+-)
  Iabc/1 -> Measurements/2(Iabc)
  Mux/1 -> m/1
  Control loops/3(m) -> Mux/1
  Pset/1 -> Control loops/1(Pset)
  Qset/1 -> Control loops/2(Qset)
  Block/1 -> Control loops/6(Block)
  Edc/1 -> Control loops/7(Edc)

== system callGAMS/sm_computation/G3/VSC v2/VSC Model ==
  Ref : Inport
  EMT AVG : Subsystem  VariantControl=EMT_AVG
  EMT SW : Subsystem  VariantControl=EMT_SW
  Phasor : Subsystem  VariantControl=Phasor
  A : PMIOPort  Side=Left
  B : PMIOPort  Port=2  Side=Left
  C : PMIOPort  Port=3  Side=Left

== system callGAMS/sm_computation/G3/VSC v2/output signals ==
  Vs : Inport
  Is : Inport  Port=2
  control : Inport  Port=3
  Bus Creator : BusCreator  Inputs=15
  Demux : Demux  Outputs=13
  m : Outport
  wires:
  Bus Creator/1 -> m/1
  control/1 -> Demux/1
  Vs/1 -> Bus Creator/1  "Vabc"
  Is/1 -> Bus Creator/2  "Iabc"
  Demux/1 -> Bus Creator/3  "vqp"
  Demux/2 -> Bus Creator/4  "vdp"
  Demux/3 -> Bus Creator/5  "vqn"
  Demux/4 -> Bus Creator/6  "vdn"
  Demux/5 -> Bus Creator/7  "iqp"
  Demux/6 -> Bus Creator/8  "idp"
  Demux/7 -> Bus Creator/9  "iqn"
  Demux/8 -> Bus Creator/10  "idn"
  Demux/9 -> Bus Creator/11  "f"
  Demux/10 -> Bus Creator/12  "Pdq"
  Demux/11 -> Bus Creator/13  "Qdq"
  Demux/12 -> Bus Creator/14  "Pabc"
  Demux/13 -> Bus Creator/15  "Qabc"

== system callGAMS/sm_computation/G5/VSC v2/VI measurement1 ==
  Current Measurement : spsCurrentMeasurementLib/Current Measurement  PhasorSimulation=on  OutputType=Complex  PSBequivalent=0
  Current Measurement1 : spsCurrentMeasurementLib/Current Measurement  PhasorSimulation=on  OutputType=Complex  PSBequivalent=0
  Current Measurement2 : spsCurrentMeasurementLib/Current Measurement  PhasorSimulation=on  OutputType=Complex  PSBequivalent=0
  Ground : spsGroundLib/Ground  LConnTagsString=a
  Ground1 : spsGroundLib/Ground  LConnTagsString=a
  Ground2 : spsGroundLib/Ground  LConnTagsString=a
  Mux : Mux  Inputs=3
  Mux1 : Mux  Inputs=3
  Voltage Measurement1 : spsVoltageMeasurementLib/Voltage Measurement  PhasorSimulation=on  OutputType=Complex  PSBequivalent=0
  Voltage Measurement2 : spsVoltageMeasurementLib/Voltage Measurement  PhasorSimulation=on  OutputType=Complex  PSBequivalent=0
  Voltage Measurement3 : spsVoltageMeasurementLib/Voltage Measurement  PhasorSimulation=on  OutputType=Complex  PSBequivalent=0
  A : PMIOPort  Side=Left
  B : PMIOPort  Port=2  Side=Left
  C : PMIOPort  Port=3  Side=Left
  a : PMIOPort  Port=4  Side=Right
  b : PMIOPort  Port=5  Side=Right
  c : PMIOPort  Port=6  Side=Right
  Vs : Outport
  Is : Outport  Port=2
  wires:
  Mux1/1 -> Is/1
  Mux/1 -> Vs/1
  Voltage Measurement1/1 -> Mux/2
  Voltage Measurement2/1 -> Mux/3
  Current Measurement2/1 -> Mux1/3
  Voltage Measurement3/1 -> Mux/1
  Current Measurement/1 -> Mux1/1
  Current Measurement1/1 -> Mux1/2
  connections:
  Voltage Measurement3/LConn1 -- A/RConn1 -- Current Measurement/LConn1
  Current Measurement2/LConn1 -- C/RConn1 -- Voltage Measurement2/LConn1
  B/RConn1 -- Voltage Measurement1/LConn1 -- Current Measurement1/LConn1
  Current Measurement1/RConn1 -- b/RConn1
  Current Measurement/RConn1 -- a/RConn1
  Current Measurement2/RConn1 -- c/RConn1
  Ground1/LConn1 -- Voltage Measurement1/LConn2
  Ground2/LConn1 -- Voltage Measurement2/LConn2
  Ground/LConn1 -- Voltage Measurement3/LConn2

== system callGAMS/sm_computation/G5/VSC v2/VSC Control ==
  Block : Inport
  Vabc : Inport  Port=2
  Iabc : Inport  Port=3
  Pset : Inport  Port=4
  Qset : Inport  Port=5
  Edc : Inport  Port=6
  Control loops : Subsystem  Variant=on  VariantControlMode=label  LabelModeActiveChoice=Phasor_I_ref
  Measurements : Subsystem  Variant=on  VariantControlMode=label  LabelModeActiveChoice=Phasor
  Modulation : Subsystem  Variant=on  VariantControlMode=label  LabelModeActiveChoice=Phasor_I_and_PQ
  Mux : Mux  Inputs=2
  Ref : Outport
  m : Outport  Port=2
  wires:
  Control loops/2(iqd+-ref) -> Modulation/3(iqd+-*)
  Control loops/1(vqd+-ref) -> Modulation/2(vqd+-*)
  [PQabc] -> Mux/2
  Measurements/5(PQabc) -> [PQabc]
  Modulation/1(Ref) -> Ref/1
  Measurements/4(theta) -> [theta]
  Vabc/1 -> Measurements/1(Vabc)
  Measurements/1(vqd+-) -> Control loops/3(vqd+-), [vqdpn]
  Measurements/2(iqd+-) -> Control loops/4(iqd+-)
  Measurements/3(freq) -> Control loops/5(freq)
  [theta] -> Modulation/4(theta)
  [vqdpn] -> Modulation/1(vqd+-)
  Iabc/1 -> Measurements/2(Iabc)
  Mux/1 -> m/1
  Control loops/3(m) -> Mux/1
  Pset/1 -> Control loops/1(Pset)
  Qset/1 -> Control loops/2(Qset)
  Block/1 -> Control loops/6(Block)
  Edc/1 -> Control loops/7(Edc)

== system callGAMS/sm_computation/G5/VSC v2/VSC Model ==
  Ref : Inport
  EMT AVG : Subsystem  VariantControl=EMT_AVG
  EMT SW : Subsystem  VariantControl=EMT_SW
  Phasor : Subsystem  VariantControl=Phasor
  A : PMIOPort  Side=Left
  B : PMIOPort  Port=2  Side=Left
  C : PMIOPort  Port=3  Side=Left

== system callGAMS/sm_computation/G5/VSC v2/output signals ==
  Vs : Inport
  Is : Inport  Port=2
  control : Inport  Port=3
  Bus Creator : BusCreator  Inputs=15
  Demux : Demux  Outputs=13
  m : Outport
  wires:
  Bus Creator/1 -> m/1
  control/1 -> Demux/1
  Vs/1 -> Bus Creator/1  "Vabc"
  Is/1 -> Bus Creator/2  "Iabc"
  Demux/1 -> Bus Creator/3  "vqp"
  Demux/2 -> Bus Creator/4  "vdp"
  Demux/3 -> Bus Creator/5  "vqn"
  Demux/4 -> Bus Creator/6  "vdn"
  Demux/5 -> Bus Creator/7  "iqp"
  Demux/6 -> Bus Creator/8  "idp"
  Demux/7 -> Bus Creator/9  "iqn"
  Demux/8 -> Bus Creator/10  "idn"
  Demux/9 -> Bus Creator/11  "f"
  Demux/10 -> Bus Creator/12  "Pdq"
  Demux/11 -> Bus Creator/13  "Qdq"
  Demux/12 -> Bus Creator/14  "Pabc"
  Demux/13 -> Bus Creator/15  "Qabc"

== system callGAMS/sm_computation/G6/VSC v2/VI measurement1 ==
  Current Measurement : spsCurrentMeasurementLib/Current Measurement  PhasorSimulation=on  OutputType=Complex  PSBequivalent=0
  Current Measurement1 : spsCurrentMeasurementLib/Current Measurement  PhasorSimulation=on  OutputType=Complex  PSBequivalent=0
  Current Measurement2 : spsCurrentMeasurementLib/Current Measurement  PhasorSimulation=on  OutputType=Complex  PSBequivalent=0
  Ground : spsGroundLib/Ground  LConnTagsString=a
  Ground1 : spsGroundLib/Ground  LConnTagsString=a
  Ground2 : spsGroundLib/Ground  LConnTagsString=a
  Mux : Mux  Inputs=3
  Mux1 : Mux  Inputs=3
  Voltage Measurement1 : spsVoltageMeasurementLib/Voltage Measurement  PhasorSimulation=on  OutputType=Complex  PSBequivalent=0
  Voltage Measurement2 : spsVoltageMeasurementLib/Voltage Measurement  PhasorSimulation=on  OutputType=Complex  PSBequivalent=0
  Voltage Measurement3 : spsVoltageMeasurementLib/Voltage Measurement  PhasorSimulation=on  OutputType=Complex  PSBequivalent=0
  A : PMIOPort  Side=Left
  B : PMIOPort  Port=2  Side=Left
  C : PMIOPort  Port=3  Side=Left
  a : PMIOPort  Port=4  Side=Right
  b : PMIOPort  Port=5  Side=Right
  c : PMIOPort  Port=6  Side=Right
  Vs : Outport
  Is : Outport  Port=2
  wires:
  Mux1/1 -> Is/1
  Mux/1 -> Vs/1
  Voltage Measurement1/1 -> Mux/2
  Voltage Measurement2/1 -> Mux/3
  Current Measurement2/1 -> Mux1/3
  Voltage Measurement3/1 -> Mux/1
  Current Measurement/1 -> Mux1/1
  Current Measurement1/1 -> Mux1/2
  connections:
  Voltage Measurement3/LConn1 -- A/RConn1 -- Current Measurement/LConn1
  Current Measurement2/LConn1 -- C/RConn1 -- Voltage Measurement2/LConn1
  B/RConn1 -- Voltage Measurement1/LConn1 -- Current Measurement1/LConn1
  Current Measurement1/RConn1 -- b/RConn1
  Current Measurement/RConn1 -- a/RConn1
  Current Measurement2/RConn1 -- c/RConn1
  Ground1/LConn1 -- Voltage Measurement1/LConn2
  Ground2/LConn1 -- Voltage Measurement2/LConn2
  Voltage Measurement3/LConn2 -- Ground/LConn1

== system callGAMS/sm_computation/G6/VSC v2/VSC Control ==
  Block : Inport
  Vabc : Inport  Port=2
  Iabc : Inport  Port=3
  Pset : Inport  Port=4
  Qset : Inport  Port=5
  Edc : Inport  Port=6
  Control loops : Subsystem  Variant=on  VariantControlMode=label  LabelModeActiveChoice=Phasor_I_ref
  Measurements : Subsystem  Variant=on  VariantControlMode=label  LabelModeActiveChoice=Phasor
  Modulation : Subsystem  Variant=on  VariantControlMode=label  LabelModeActiveChoice=Phasor_I_and_PQ
  Mux : Mux  Inputs=2
  Ref : Outport
  m : Outport  Port=2
  wires:
  Control loops/2(iqd+-ref) -> Modulation/3(iqd+-*)
  Control loops/1(vqd+-ref) -> Modulation/2(vqd+-*)
  [PQabc] -> Mux/2
  Measurements/5(PQabc) -> [PQabc]
  Modulation/1(Ref) -> Ref/1
  Measurements/4(theta) -> [theta]
  Vabc/1 -> Measurements/1(Vabc)
  Measurements/1(vqd+-) -> Control loops/3(vqd+-), [vqdpn]
  Measurements/2(iqd+-) -> Control loops/4(iqd+-)
  Measurements/3(freq) -> Control loops/5(freq)
  [theta] -> Modulation/4(theta)
  [vqdpn] -> Modulation/1(vqd+-)
  Iabc/1 -> Measurements/2(Iabc)
  Mux/1 -> m/1
  Control loops/3(m) -> Mux/1
  Pset/1 -> Control loops/1(Pset)
  Qset/1 -> Control loops/2(Qset)
  Block/1 -> Control loops/6(Block)
  Edc/1 -> Control loops/7(Edc)

== system callGAMS/sm_computation/G6/VSC v2/VSC Model ==
  Ref : Inport
  EMT AVG : Subsystem  VariantControl=EMT_AVG
  EMT SW : Subsystem  VariantControl=EMT_SW
  Phasor : Subsystem  VariantControl=Phasor
  A : PMIOPort  Side=Left
  B : PMIOPort  Port=2  Side=Left
  C : PMIOPort  Port=3  Side=Left

== system callGAMS/sm_computation/G6/VSC v2/output signals ==
  Vs : Inport
  Is : Inport  Port=2
  control : Inport  Port=3
  Bus Creator : BusCreator  Inputs=15
  Demux : Demux  Outputs=13
  m : Outport
  wires:
  Bus Creator/1 -> m/1
  control/1 -> Demux/1
  Vs/1 -> Bus Creator/1  "Vabc"
  Is/1 -> Bus Creator/2  "Iabc"
  Demux/1 -> Bus Creator/3  "vqp"
  Demux/2 -> Bus Creator/4  "vdp"
  Demux/3 -> Bus Creator/5  "vqn"
  Demux/4 -> Bus Creator/6  "vdn"
  Demux/5 -> Bus Creator/7  "iqp"
  Demux/6 -> Bus Creator/8  "idp"
  Demux/7 -> Bus Creator/9  "iqn"
  Demux/8 -> Bus Creator/10  "idn"
  Demux/9 -> Bus Creator/11  "f"
  Demux/10 -> Bus Creator/12  "Pdq"
  Demux/11 -> Bus Creator/13  "Qdq"
  Demux/12 -> Bus Creator/14  "Pabc"
  Demux/13 -> Bus Creator/15  "Qabc"
